simulink model "SecOrdMdl_Initial"  (R2023b)
settings: Solver=ode8  StartTime=0.0  StopTime=5  FixedStep=1e-3  RelTol=1e-3
values from neighbouring files (symbols this model uses):
  A = [getAerodynamics(x0(1)*1/Ng,x0(2),v_arr(i))/(J*x0(1)^2)-Dg/J 0 ... (first row only)    [LQR_GAINSCHEDULING.m]    (also in SecondOrderModel.m = [getAerodynamics(x0(1)*1/Ng,x0(2),v)/(J*x0(1)^2)-Dg/J 0)
  B = [Dg*omega_0/(J*p*x0(2)); 1/tau_theta]    [LQR_GAINSCHEDULING.m]    (also in SecondOrderModel.m)
  C = diag([1 1])    [SecondOrderModel.m]
  J = Jr/(Ng^2) + Jg    [SecondOrderModel.m]
  k0 = p_aer(:,3)    [SecondOrderModel.m]
  k1 = p_aer(:,2)    [SecondOrderModel.m]
  k2 = p_aer(:,1)    [SecondOrderModel.m]
  Tg = Dg*s    [SecondOrderModel.m]
  x0 = [omega_g0; u0]    [SecondOrderModel.m]
undefined symbols (not defined in the file or in its folder): Dg, Ng, omega_0, omega_g0, p, tau_theta, theta_dot_max, theta_max, theta_min
libraries: slpidlib x1, cstblocks x1, simulink x1
settings Model: Creator=Selim  LastModifiedBy=Selim

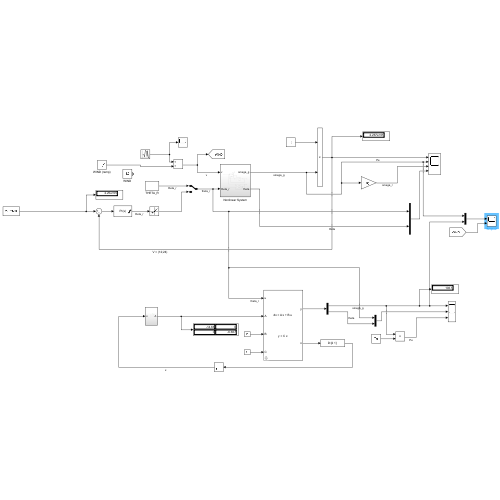
[thumbnail: Simulink's stored preview of the top-level diagram]
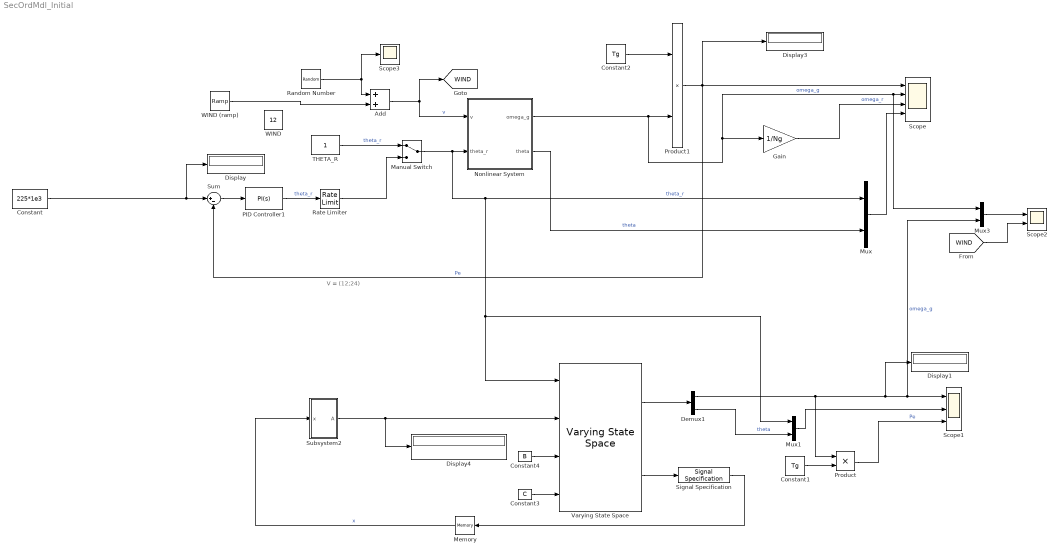
== system SecOrdMdl_Initial ==
  note: V = (12;24)
  Add : Sum
  Constant : Constant  Value=225*1e3
  Constant1 : Constant  Value=Tg
  Constant2 : Constant  Value=Tg
  Constant3 : Constant  Value=C
  Constant4 : Constant  Value=B
  Demux1 : Demux  Outputs=2
  Display{,1,3..4} (4 alike) : Display
  Gain : Gain  Gain=1/Ng
  Manual Switch : ManualSwitch
  Memory : Memory  InitialCondition=x0
  Mux : Mux  Inputs=2
  Mux1 : Mux  Inputs=2
  Mux3 : Mux  Inputs=2
  Nonlinear System : Subsystem
  PID Controller1 : slpidlib/PID Controller  Controller=PI  Form=Parallel  TimeDomain=Continuous-time  UseExternalTs=off  SampleTime=-1  IntegratorMethod=Forward Euler  FilterMethod=Forward Euler  ControllerParametersSource=internal  P=-6.03660291875363e-05  I=-0.00249732862255308  UseKiTs=off  D=-0.00034354310668366  N=1044.45037459015  UseFilter=on  TunerSelectOption=Transfer Function Based (PID Tuner App)  InitialConditionSource=internal  InitialConditionForIntegrator=0  InitialConditionForFilter=0  DifferentiatorICPrevScaledInput=0  ExternalReset=none  TrackingMode=off  Kt=1  LimitOutput=on  SatLimitsSource=internal  UpperSaturationLimit=theta_max  LowerSaturationLimit=theta_min  LinearizeAsGain=on  AntiWindupMode=clamping  Kb=1  LimitIntegrator=off  UpperIntegratorSaturationLimit=inf  LowerIntegratorSaturationLimit=-inf  POutMin=[]  POutMax=[]  IOutMin=[]  IOutMax=[]  DOutMin=[]  DOutMax=[]  NOutMin=[]  NOutMax=[]  SumOutMin=[]  SumOutMax=[]  SaturationOutMin=[]  SaturationOutMax=[]  PParamMin=[]  PParamMax=[]  IParamMin=[]  IParamMax=[]  DParamMin=[]  DParamMax=[]  NParamMin=[]  NParamMax=[]  KbParamMin=[]  KbParamMax=[]  KtParamMin=[]  KtParamMax=[]  KbOutMin=[]  KbOutMax=[]  KtOutMin=[]  KtOutMax=[]  IntegratorOutMin=[]  IntegratorOutMax=[]  FilterOutMin=[]  FilterOutMax=[]  SumI1OutMin=[]  SumI1OutMax=[]  SumI2OutMin=[]  SumI2OutMax=[]  SumI3OutMin=[]  SumI3OutMax=[]  SumI4OutMin=[]  SumI4OutMax=[]  SumDOutMin=[]  SumDOutMax=[]  DifferentiatorOutMin=[]  DifferentiatorOutMax=[]  FilterDiffOutCoefMin=[]  FilterDiffOutCoefMax=[]  ReciprocalOutMin=[]  ReciprocalOutMax=[]  SumDenOutMin=[]  SumDenOutMax=[]  SumNumOutMin=[]  SumNumOutMax=[]  DivideOutMin=[]  DivideOutMax=[]  UdiffTsProdOutMin=[]  UdiffTsProdOutMax=[]  NTsProdOutMin=[]  NTsProdOutMax=[]  UintegralTsProdOutMin=[]  UintegralTsProdOutMax=[]  UngainTsProdOutMin=[]  UngainTsProdOutMax=[]  ClampingZeroOutDataTypeStr=Inherit: Inherit via back propagation  ClampingZeroOutMin=[]  ClampingZeroOutMax=[]  FilterDenConstantOutDataTypeStr=Inherit: Inherit via back propagation  FilterDenConstantOutMin=[]  FilterDenConstantOutMax=[]  PCopyOutDataTypeStr=Inherit: Inherit via back propagation  PCopyOutMin=[]  PCopyOutMax=[]  NCopyOutDataTypeStr=Inherit: Inherit via back propagation  NCopyOutMin=[]  NCopyOutMax=[]  IntegratorContinuousStateAttributes=''  IntegratorStateMustResolveToSignalObject=off  IntegratorRTWStateStorageClass=Auto  FilterContinuousStateAttributes=''  FilterStateMustResolveToSignalObject=off  FilterRTWStateStorageClass=Auto  ParallelPVariant=InternalParameters  IdealPVariant=Disabled  IVariant=InternalParameters  DVariant=Disabled  IntegratorVariant=Continuous  SatVariant=Enabled  AWVariant=ContClampingParallel  PCopyVariant=Disabled  TRVariant=Disabled  FdbkBlocksVariant=Forward  IdealPFdbkVariant=Disabled  SatFdbkVariant=Disabled  DerivativeFilterVariant=Disabled  NVariant=Disabled  NCopyVariant=Disabled_SignalSpec  FilterICVariant=Disabled  IntegratorICVariant=InternalICs  ExternalResetVariant=Disabled  TRSumVariant=Passthrough  SumFdbkVariant=Disabled  SumVariant=Sum_PI  TsampFilterVariant=InternalTs  TsampNgainVariant=Passthrough  TsampIntegralVariant=Disabled_SignalSpec  ExternalSaturationOutDataTypeStr=Inherit: Same as second input
  Product : Product
  Product1 : Product
  Random Number : RandomNumber  Variance=5  SampleTime=1e-2
  Rate Limiter : RateLimiter  RisingSlewLimit=theta_dot_max  FallingSlewLimit=-theta_dot_max  SampleTimeMode=inherited
  Scope : Scope  NumInputPorts=4
  Scope1 : Scope  NumInputPorts=3
  Scope2 : Scope  NumInputPorts=2
  Scope3 : Scope
  Signal Specification : SignalSpecification  Dimensions=[2 1]
  Subsystem2 : Subsystem
  Sum : Sum  Inputs=|+-
  THETA_R : Constant
  Varying State Space : cstblocks/Linear Parameter Varying/Varying State Space  x0=x0  xNames=''  OutputX=on  OutputDX=off  Feedthrough=off
  WIND : Constant  Value=12
  WIND (ramp) : simulink/Sources/Ramp  slope=2  start=1  InitialOutput=12
  tag scope: WIND=global
  wires:
  Add/1 -> Nonlinear System/1(v), [WIND]  "v"
  PID Controller1/1 -> Rate Limiter/1  "theta_r"
  Nonlinear System/2(theta) -> Mux/2  "theta"
  Nonlinear System/1(omega_g) -> Mux3/1, Scope/2, Gain/1, Product1/2  "omega_g"
  Product1/1 -> Sum/2, Display3/1, Scope/1  "Pe"
  Sum/1 -> PID Controller1/1
  Constant/1 -> Display/1, Sum/1
  THETA_R/1 -> Manual Switch/1  "theta_r"
  Manual Switch/1 -> Mux/1, Varying State Space/1, Mux1/1, Nonlinear System/2(theta_r)  "theta_r"
  Constant2/1 -> Product1/1
  Gain/1 -> Scope/3  "omega_r"
  Mux/1 -> Scope/4
  Constant3/1 -> Varying State Space/4
  Constant4/1 -> Varying State Space/3
  Varying State Space/2 -> Signal Specification/1
  Signal Specification/1 -> Memory/1
  Varying State Space/1 -> Demux1/1
  Demux1/1 -> Display1/1, Mux3/2, Scope1/1, Product/1  "omega_g"
  Demux1/2 -> Mux1/2  "theta"
  Rate Limiter/1 -> Manual Switch/2
  Memory/1 -> Subsystem2/1(x)  "x"
  Mux1/1 -> Scope1/2
  Constant1/1 -> Product/2
  Product/1 -> Scope1/3  "Pe"
  Subsystem2/1(A) -> Display4/1, Varying State Space/2
  Mux3/1 -> Scope2/1
  Random Number/1 -> Scope3/1, Add/1
  WIND (ramp)/1 -> Add/2
  [WIND] -> Scope2/2

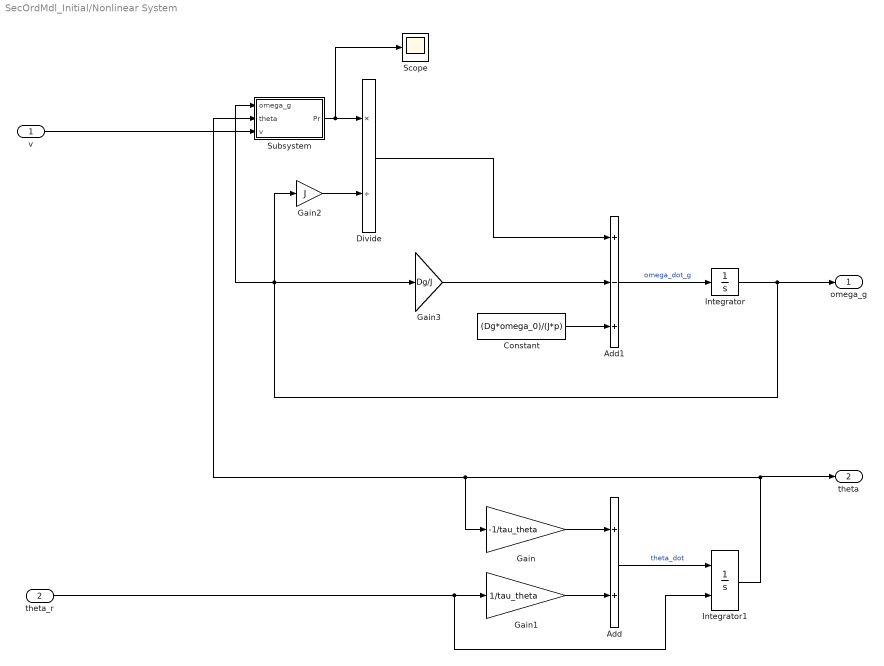
== system SecOrdMdl_Initial/Nonlinear System ==
  v : Inport
  theta_r : Inport  Port=2
  Add : Sum
  Add1 : Sum  Inputs=+-+
  Constant : Constant  Value=(Dg*omega_0)/(J*p)
  Divide : Product  Inputs=*/
  Gain : Gain  Gain=-1/tau_theta
  Gain1 : Gain  Gain=1/tau_theta
  Gain2 : Gain  Gain=J
  Gain3 : Gain  Gain=Dg/J
  Integrator : Integrator  InitialCondition=x0(1)
  Integrator1 : Integrator  InitialConditionSource=external  InitialCondition=1
  Scope : Scope
  Subsystem : Subsystem
  omega_g : Outport
  theta : Outport  Port=2
  wires:
  Gain3/1 -> Add1/2
  Integrator/1 -> Subsystem/1(omega_g), Gain3/1, Gain2/1, omega_g/1
  Integrator1/1 -> Subsystem/2(theta), Gain/1, theta/1
  Constant/1 -> Add1/3
  Gain/1 -> Add/1
  Subsystem/1(Pr) -> Scope/1, Divide/1
  Gain1/1 -> Add/2
  Gain2/1 -> Divide/2
  Divide/1 -> Add1/1
  v/1 -> Subsystem/3(v)
  Add1/1 -> Integrator/1  "omega_dot_g"
  Add/1 -> Integrator1/1  "theta_dot"
  theta_r/1 -> Integrator1/2, Gain1/1

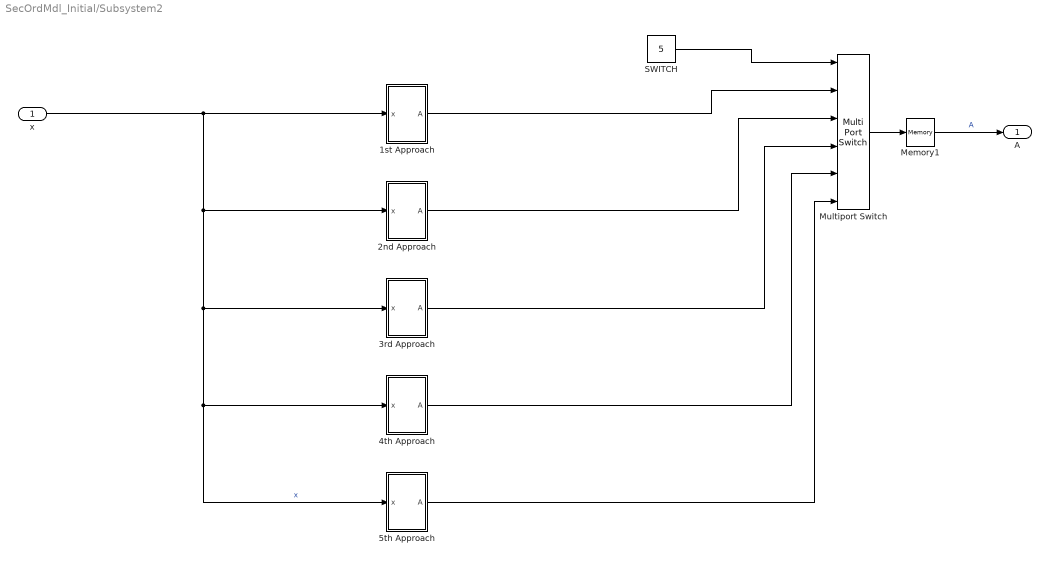
== system SecOrdMdl_Initial/Subsystem2 ==
  x : Inport
  1st Approach : Subsystem
  2nd Approach : Subsystem
  3rd Approach : Subsystem
  4th Approach : Subsystem
  5th Approach : Subsystem
  Memory1 : Memory  InitialCondition=A
  Multiport Switch : MultiPortSwitch  Inputs=5  SaturateOnIntegerOverflow=off  InputSameDT=off
  SWITCH : Constant  Value=5
  A : Outport
  wires:
  Memory1/1 -> A/1  "A"
  x/1 -> 5th Approach/1(x), 4th Approach/1(x), 3rd Approach/1(x), 2nd Approach/1(x), 1st Approach/1(x)  "x"
  1st Approach/1(A) -> Multiport Switch/2
  Multiport Switch/1 -> Memory1/1
  2nd Approach/1(A) -> Multiport Switch/3
  3rd Approach/1(A) -> Multiport Switch/4
  SWITCH/1 -> Multiport Switch/1
  4th Approach/1(A) -> Multiport Switch/5
  5th Approach/1(A) -> Multiport Switch/6

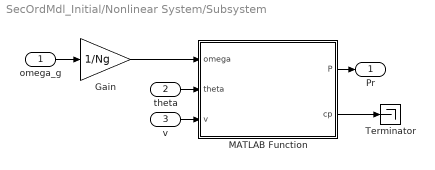
== system SecOrdMdl_Initial/Nonlinear System/Subsystem ==
  omega_g : Inport
  theta : Inport  Port=2
  v : Inport  Port=3
  Gain : Gain  Gain=1/Ng
  MATLAB Function : MATLAB Function  TreatAsAtomicUnit=on
  Terminator : Terminator
  Pr : Outport
  wires:
  theta/1 -> MATLAB Function/2(theta)
  MATLAB Function/2(cp) -> Terminator/1
  MATLAB Function/1(P) -> Pr/1
  v/1 -> MATLAB Function/3(v)
  omega_g/1 -> Gain/1
  Gain/1 -> MATLAB Function/1(omega)

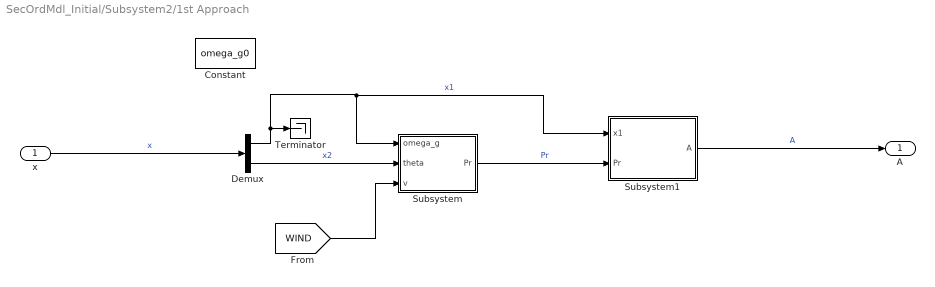
== system SecOrdMdl_Initial/Subsystem2/1st Approach ==
  x : Inport
  Constant : Constant  Value=omega_g0
  Demux : Demux  Outputs=2
  Subsystem : Subsystem
  Subsystem1 : Subsystem
  Terminator : Terminator
  A : Outport
  wires:
  Demux/2 -> Subsystem/2(theta)  "x2"
  Subsystem/1(Pr) -> Subsystem1/2(Pr)  "Pr"
  Subsystem1/1(A) -> A/1  "A"
  Demux/1 -> Subsystem1/1(x1), Subsystem/1(omega_g), Terminator/1  "x1"
  [WIND] -> Subsystem/3(v)
  x/1 -> Demux/1  "x"

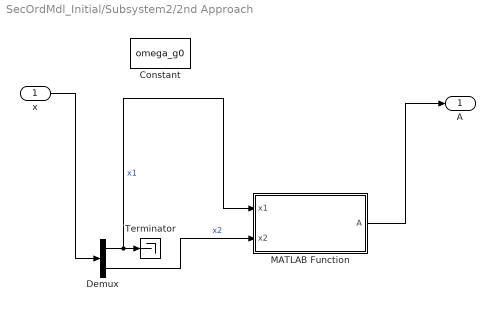
== system SecOrdMdl_Initial/Subsystem2/2nd Approach ==
  x : Inport
  Constant : Constant  Value=omega_g0
  Demux : Demux  Outputs=2
  MATLAB Function : MATLAB Function  TreatAsAtomicUnit=on
  Terminator : Terminator
  A : Outport
  wires:
  Demux/1 -> MATLAB Function/1(x1), Terminator/1  "x1"
  MATLAB Function/1(A) -> A/1
  Demux/2 -> MATLAB Function/2(x2)  "x2"
  x/1 -> Demux/1

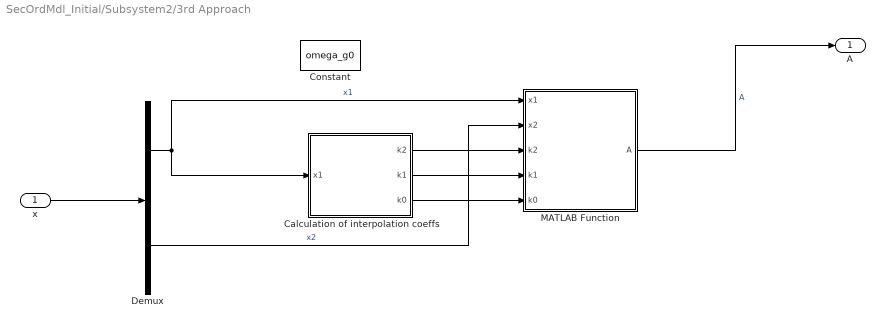
== system SecOrdMdl_Initial/Subsystem2/3rd Approach ==
  x : Inport
  Calculation of interpolation coeffs : Subsystem
  Constant : Constant  Value=omega_g0
  Demux : Demux  Outputs=2
  MATLAB Function : MATLAB Function  TreatAsAtomicUnit=on
  A : Outport
  wires:
  Calculation of interpolation coeffs/1(k2) -> MATLAB Function/3(k2)
  MATLAB Function/1(A) -> A/1  "A"
  Demux/2 -> MATLAB Function/2(x2)  "x2"
  Calculation of interpolation coeffs/2(k1) -> MATLAB Function/4(k1)
  Demux/1 -> MATLAB Function/1(x1), Calculation of interpolation coeffs/1(x1)  "x1"
  Calculation of interpolation coeffs/3(k0) -> MATLAB Function/5(k0)
  x/1 -> Demux/1

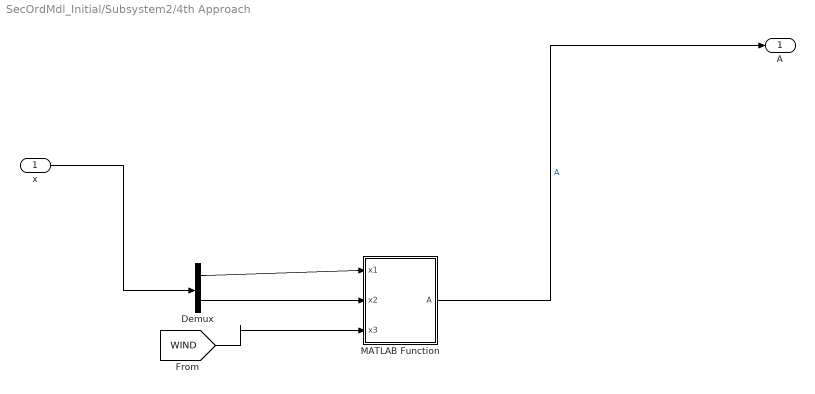
== system SecOrdMdl_Initial/Subsystem2/4th Approach ==
  x : Inport
  Demux : Demux  Outputs=2
  MATLAB Function : MATLAB Function  TreatAsAtomicUnit=on
  A : Outport
  wires:
  Demux/2 -> MATLAB Function/2(x2)
  [WIND] -> MATLAB Function/3(x3)
  Demux/1 -> MATLAB Function/1(x1)
  MATLAB Function/1(A) -> A/1  "A"
  x/1 -> Demux/1

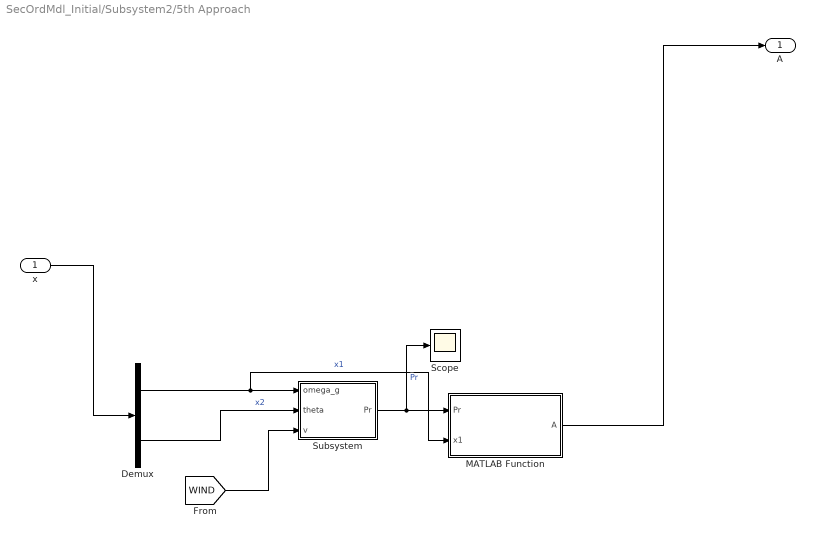
== system SecOrdMdl_Initial/Subsystem2/5th Approach ==
  x : Inport
  Demux : Demux  Outputs=2
  MATLAB Function : MATLAB Function  TreatAsAtomicUnit=on
  Scope : Scope
  Subsystem : Subsystem
  A : Outport
  wires:
  x/1 -> Demux/1
  Demux/2 -> Subsystem/2(theta)  "x2"
  [WIND] -> Subsystem/3(v)
  Subsystem/1(Pr) -> Scope/1, MATLAB Function/1(Pr)  "Pr"
  MATLAB Function/1(A) -> A/1
  Demux/1 -> MATLAB Function/2(x1), Subsystem/1(omega_g)  "x1"

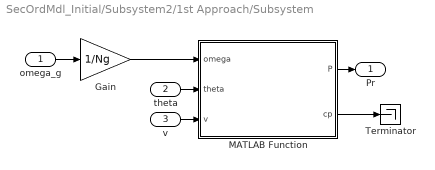
== system SecOrdMdl_Initial/Subsystem2/1st Approach/Subsystem ==
  omega_g : Inport
  theta : Inport  Port=2
  v : Inport  Port=3
  Gain : Gain  Gain=1/Ng
  MATLAB Function : MATLAB Function  TreatAsAtomicUnit=on
  Terminator : Terminator
  Pr : Outport
  wires:
  theta/1 -> MATLAB Function/2(theta)
  MATLAB Function/2(cp) -> Terminator/1
  MATLAB Function/1(P) -> Pr/1
  v/1 -> MATLAB Function/3(v)
  omega_g/1 -> Gain/1
  Gain/1 -> MATLAB Function/1(omega)

== system SecOrdMdl_Initial/Subsystem2/1st Approach/Subsystem1 ==
  x1 : Inport
  Pr : Inport  Port=2
  MATLAB Function : MATLAB Function  TreatAsAtomicUnit=on
  A : Outport
  wires:
  Pr/1 -> MATLAB Function/2(Pr)
  MATLAB Function/1(A) -> A/1  "A"
  x1/1 -> MATLAB Function/1(x1)

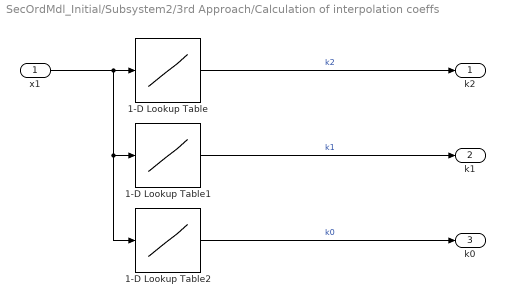
== system SecOrdMdl_Initial/Subsystem2/3rd Approach/Calculation of interpolation coeffs ==
  x1 : Inport
  1-D Lookup Table : Lookup_n-D  NumberOfTableDimensions=1  BreakpointsForDimension1=omega_g_arr'  Table=k2  InternalRulePriority=Speed  RndMeth=Simplest
  1-D Lookup Table1 : Lookup_n-D  NumberOfTableDimensions=1  BreakpointsForDimension1=omega_g_arr'  Table=k1  InternalRulePriority=Speed  RndMeth=Simplest
  1-D Lookup Table2 : Lookup_n-D  NumberOfTableDimensions=1  BreakpointsForDimension1=omega_g_arr'  Table=k0  InternalRulePriority=Speed  RndMeth=Simplest
  k2 : Outport
  k1 : Outport  Port=2
  k0 : Outport  Port=3
  wires:
  x1/1 -> 1-D Lookup Table2/1, 1-D Lookup Table1/1, 1-D Lookup Table/1
  1-D Lookup Table/1 -> k2/1  "k2"
  1-D Lookup Table2/1 -> k0/1  "k0"
  1-D Lookup Table1/1 -> k1/1  "k1"

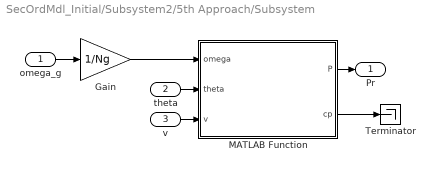
== system SecOrdMdl_Initial/Subsystem2/5th Approach/Subsystem ==
  omega_g : Inport
  theta : Inport  Port=2
  v : Inport  Port=3
  Gain : Gain  Gain=1/Ng
  MATLAB Function : MATLAB Function  TreatAsAtomicUnit=on
  Terminator : Terminator
  Pr : Outport
  wires:
  theta/1 -> MATLAB Function/2(theta)
  MATLAB Function/2(cp) -> Terminator/1
  MATLAB Function/1(P) -> Pr/1
  v/1 -> MATLAB Function/3(v)
  omega_g/1 -> Gain/1
  Gain/1 -> MATLAB Function/1(omega)

== matlab function SecOrdMdl_Initial/Subsystem2/1st Approach/Subsystem1/MATLAB Function ==
  data: x1 input; A output; J parameter; Dg parameter; Pr input; tau_theta parameter
function A = getMatrixA(x1,J,Dg,Pr,tau_theta)

Kx1 = -Pr/(J*x1^2) - Dg/J;

A = [Kx1 0; 0 -1/tau_theta];

== matlab function SecOrdMdl_Initial/Nonlinear System/Subsystem/MATLAB Function ==
  data: omega input; P output; theta input; v input; cp output
function [P,cp] = getAerodynamics(omega,theta,v)

R = 14.5;
rho = 1.2;

lambda = v/(R*omega);
lambda_t = 1/(1/(lambda^-1 + 0.12*theta) - 0.0035/((1.5*theta)^3 + 1));

cp = 0.22*(116/lambda_t - 0.6*theta - 5)*exp(-12.5/lambda_t);

P = 1/2*rho*pi*(R^2)*(v^3)*cp;

== matlab function SecOrdMdl_Initial/Subsystem2/1st Approach/Subsystem/MATLAB Function ==
  data: omega input; P output; theta input; v input; cp output
function [P,cp] = getAerodynamics(omega,theta,v)

R = 14.5;
rho = 1.2;

lambda = v/(R*omega);
lambda_t = 1/(1/(lambda^-1 + 0.12*theta) - 0.0035/((1.5*theta)^3 + 1));

cp = 0.22*(116/lambda_t - 0.6*theta - 5)*exp(-12.5/lambda_t);

P = 1/2*rho*pi*(R^2)*(v^3)*cp;

== matlab function SecOrdMdl_Initial/Subsystem2/2nd Approach/MATLAB Function ==
  data: x1 input; A output; x2 input; J parameter; Dg parameter; tau_theta parameter
function A = getMatrixA(x1,x2,J, Dg, tau_theta)

p = [-578.851267577174	-2721.27145157738	236988.438529495];

a11 = - polyval(p,x2)/(J*x1^2) - Dg/J;
a12 = (2*p(1)*x2 + p(2))/(J*x1);

A = [a11 a12; 0 -1/tau_theta];

== matlab function SecOrdMdl_Initial/Subsystem2/3rd Approach/MATLAB Function ==
  data: x1 input; A output; x2 input; k2 input; k1 input; k0 input; J parameter; Dg parameter; tau_theta parameter
function A = getMatrixA(x1,x2,k2,k1,k0,J,Dg,tau_theta)

p = [k2	k1 k0];

a11 = - polyval(p,x2)/(J*x1^2) - Dg/J;
a12 = (2*p(1)*x2 + p(2))/(J*x1);

A = [a11 a12; 0 -1/tau_theta];

== matlab function SecOrdMdl_Initial/Subsystem2/4th Approach/MATLAB Function ==
  data: x1 input; A output; x2 input; x3 input; tau_theta parameter
function A = getMatrixA(x1,x2,x3,tau_theta)

Kx1 = (7397514231676928*x3^3*pi*exp(7/(160*((27*x2^3)/8 + 1)) - 25/(2*((3*x2)/25 + (29*x1)/(2*x3))))*((33*x2)/250 - 638/(25*((3*x2)/25 + (29*x1)/(2*x3))) + 2233/(25000*((27*x2^3)/8 + 1)) + 11/10))/(9307497835634805*x1^2) - (68434404157243260928*x3^2*pi*exp(7/(160*((27*x2^3)/8 + 1)) - 25/(2*((3*x2)/25 + (29*x1)/(2*x3)))))/(232687445890870125*x1*((3*x2)/25 + (29*x1)/(2*x3))^2) - (268159890898288640*x3^2*pi*exp(7/(160*((27*x2^3)/8 + 1)) - 25/(2*((3*x2)/25 + (29*x1)/(2*x3))))*((33*x2)/250 - 638/(25*((3*x2)/25 + (29*x1)/(2*x3))) + 2233/(25000*((27*x2^3)/8 + 1)) + 11/10))/(1861499567126961*x1*((3*x2)/25 + (29*x1)/(2*x3))^2) - 83211039990087680/5584498701380883;
Kx2 = (7397514231676928*x3^3*pi*exp(7/(160*((27*x2^3)/8 + 1)) - 25/(2*((3*x2)/25 + (29*x1)/(2*x3))))*((567*x2^2)/(1280*((27*x2^3)/8 + 1)^2) - 3/(2*((3*x2)/25 + (29*x1)/(2*x3))^2))*((33*x2)/250 - 638/(25*((3*x2)/25 + (29*x1)/(2*x3))) + 2233/(25000*((27*x2^3)/8 + 1)) + 11/10))/(9307497835634805*x1) - (7397514231676928*x3^3*pi*exp(7/(160*((27*x2^3)/8 + 1)) - 25/(2*((3*x2)/25 + (29*x1)/(2*x3))))*(1914/(625*((3*x2)/25 + (29*x1)/(2*x3))^2) - (180873*x2^2)/(200000*((27*x2^3)/8 + 1)^2) + 33/250))/(9307497835634805*x1);

A = [Kx1 Kx2; 0 -1/tau_theta];

== matlab function SecOrdMdl_Initial/Subsystem2/5th Approach/MATLAB Function ==
  data: Pr input; A output; x1 input; Dg parameter; J parameter; tau_theta parameter
function A = getMatrixA(Pr,x1,Dg, J, tau_theta)

A = [Pr/(J*(x1^2))-Dg/J 0;
     0 -1/tau_theta];

== matlab function SecOrdMdl_Initial/Subsystem2/5th Approach/Subsystem/MATLAB Function ==
  data: omega input; P output; theta input; v input; cp output
function [P,cp] = getAerodynamics(omega,theta,v)

R = 14.5;
rho = 1.2;

lambda = v/(R*omega);
lambda_t = 1/(1/(lambda^-1 + 0.12*theta) - 0.0035/((1.5*theta)^3 + 1));

cp = 0.22*(116/lambda_t - 0.6*theta - 5)*exp(-12.5/lambda_t);

P = 1/2*rho*pi*(R^2)*(v^3)*cp;
